simulink model "schemf_for_4and5"  (R2021b)
settings: Solver=VariableStepAuto  StartTime=0.0  StopTime=10.0  RelTol=1e-3
values from neighbouring files (symbols this model uses):
  A = [2 6; 1 0]    [T3.m]
  B = [4; 1]    [T3.m]
  C = [2 0]    [T3.m]
  D = 6    [T3.m]
  K = -H*M0^-1    [T3.m]
  L = double([sol.l1; sol.l2])    [T3.m]
settings Model: Creator=yan  LastModifiedBy=yan

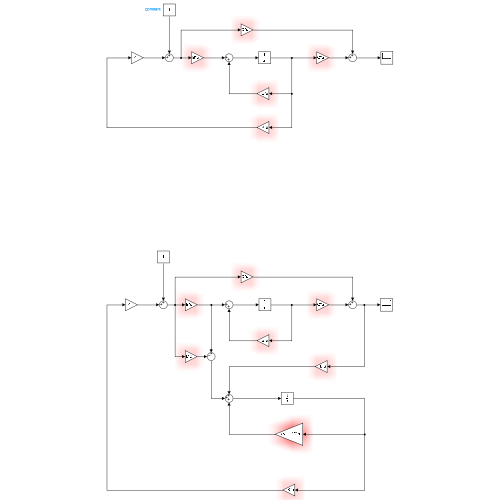
[thumbnail: Simulink's stored preview of the top-level diagram]
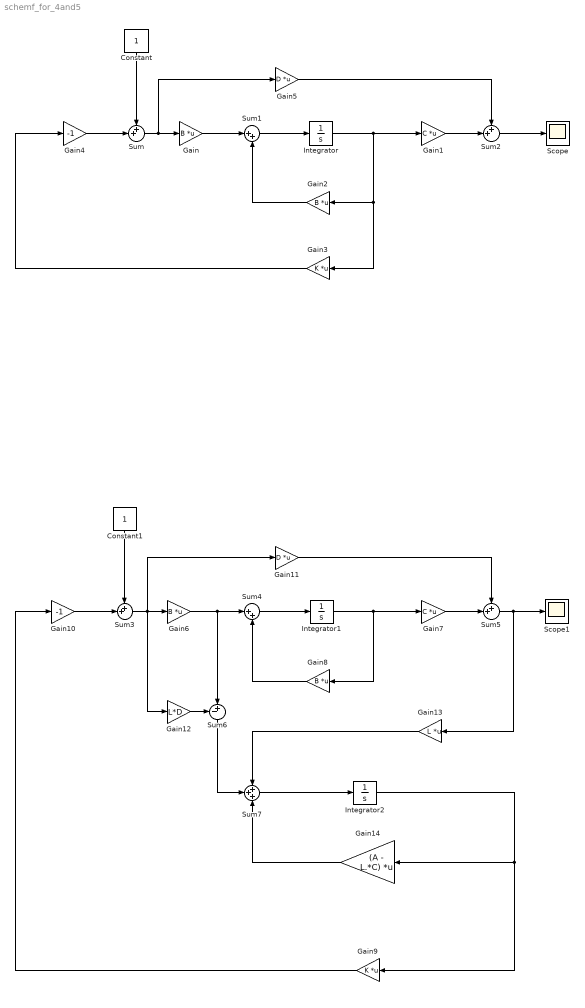
== system schemf_for_4and5 ==
  Constant : Constant
  Constant1 : Constant
  Gain{,2,6,8} (4 alike) : Gain  Gain=B  Multiplication=Matrix(K*u)
  Gain1 : Gain  Gain=C  Multiplication=Matrix(K*u)
  Gain10 : Gain  Gain=-1
  Gain11 : Gain  Gain=D  Multiplication=Matrix(K*u)
  Gain12 : Gain  Gain=L*D
  Gain13 : Gain  Gain=L  Multiplication=Matrix(K*u)
  Gain14 : Gain  Gain=(A - L.*C)  Multiplication=Matrix(K*u)
  Gain3 : Gain  Gain=K  Multiplication=Matrix(K*u)
  Gain4 : Gain  Gain=-1
  Gain5 : Gain  Gain=D  Multiplication=Matrix(K*u)
  Gain7 : Gain  Gain=C  Multiplication=Matrix(K*u)
  Gain9 : Gain  Gain=K  Multiplication=Matrix(K*u)
  Integrator : Integrator
  Integrator1 : Integrator
  Integrator2 : Integrator
  Scope : Scope
  Scope1 : Scope
  Sum{,2..3,5} (4 alike) : Sum  Inputs=++|
  Sum1 : Sum  Inputs=|++
  Sum4 : Sum  Inputs=|++
  Sum6 : Sum  Inputs=-+|
  Sum7 : Sum  Inputs=+++
  wires:
  Gain/1 -> Sum1/1
  Sum1/1 -> Integrator/1
  Integrator/1 -> Gain3/1, Gain2/1, Gain1/1
  Gain1/1 -> Sum2/2
  Constant/1 -> Sum/1
  Sum/1 -> Gain5/1, Gain/1
  Gain3/1 -> Gain4/1
  Gain2/1 -> Sum1/2
  Gain4/1 -> Sum/2
  Gain5/1 -> Sum2/1
  Sum2/1 -> Scope/1
  Gain11/1 -> Sum5/1
  Sum5/1 -> Gain13/1, Scope1/1
  Sum3/1 -> Gain12/1, Gain11/1, Gain6/1
  Sum4/1 -> Integrator1/1
  Gain6/1 -> Sum4/1, Sum6/2
  Gain8/1 -> Sum4/2
  Integrator1/1 -> Gain8/1, Gain7/1
  Gain9/1 -> Gain10/1
  Gain7/1 -> Sum5/2
  Constant1/1 -> Sum3/1
  Gain10/1 -> Sum3/2
  Gain12/1 -> Sum6/1
  Sum6/1 -> Sum7/2
  Gain13/1 -> Sum7/1
  Sum7/1 -> Integrator2/1
  Integrator2/1 -> Gain9/1, Gain14/1
  Gain14/1 -> Sum7/3
